simulink model "AccTarSel"  (R2018b)
settings: Solver=FixedStepDiscrete  StartTime=0.0  StopTime=inf  FixedStep=0.01  RelTol=1e-3
PostLoadFcn:
  | if any(exist('dsrtsu_mdlpostloadfcn', 'file') ~= 0), dsrtsu_mdlpostloadfcn('Execute', bdroot); end
values from neighbouring files (symbols this model uses):
  P_adtMaxBDC = 1.0    [AccTarSel.sldd]
  P_aFOCApproachIntpAcitve = -0.6    [AccTarSel.sldd]
  P_aFOCApproachIntpEnsure = -1.8    [AccTarSel.sldd]
  P_CutInEnable = 1.0    [AccTarSel.sldd]
  P_dAimMin = 4.5    [AccTarSel.sldd]
  P_dAimMinAVP = 1.5    [AccTarSel.sldd]
  P_dObjDrvOffMax = 5.0    [AccTarSel.sldd]
  P_dObjDrvOffMin = 3.0    [AccTarSel.sldd]
  P_dObjLowHystDecToStop = 4.5    [AccTarSel.sldd]
  P_dObjLowHystDecToStopAVP = 1.5    [AccTarSel.sldd]
  P_dObjUpperHystDecToStop = 5.0    [AccTarSel.sldd]
  P_dResMax = 5.0    [AccTarSel.sldd]
  P_dStandStill = 3.0    [AccTarSel.sldd]
  P_dStandStillMin = 2.0    [AccTarSel.sldd]
  P_dvarYMax4PO = 1.0    [AccTarSel.sldd]
  P_dyCutInThres = 3.6    [AccTarSel.sldd]
  P_facBDCInit = 0.7    [AccTarSel.sldd]
  P_facBDCIterCalc = 0.8    [AccTarSel.sldd]
  P_facFOCNegDiff = 0.3    [AccTarSel.sldd]
  P_facFOCPosDiff = 0.2    [AccTarSel.sldd]
  P_kapHystThres = 0.0005    [AccTarSel.sldd]
  P_PlausIntegDisable = 0.0    [AccTarSel.sldd]
  P_plausMin4PO = 0.5    [AccTarSel.sldd]
  P_probExistMin4PO = 0.8    [AccTarSel.sldd]
  P_StandObjEnable = 0.0    [AccTarSel.sldd]
  P_tAxTrackNegLower = 0.3    [AccTarSel.sldd]
  P_tAxTrackNegUpper = 0.6    [AccTarSel.sldd]
  P_tAxTrackPosLower = 1.0    [AccTarSel.sldd]
  P_tAxTrackPosUpper = 2.0    [AccTarSel.sldd]
  P_tBDCStartFilt = 0.2    [AccTarSel.sldd]
  P_tCSC = 3.5    [AccTarSel.sldd]
  P_tCurvFilt = 0.2    [AccTarSel.sldd]
  P_tCutInFilt = 0.5    [AccTarSel.sldd]
  P_tFiltAxAbsPONegFast = 0.1    [AccTarSel.sldd]
  P_tFiltAxAbsPONegSlow = 0.4    [AccTarSel.sldd]
  P_tFiltAxAbsPOPosFast = 1.2    [AccTarSel.sldd]
  P_tFiltAxAbsPOPosSlow = 2.0    [AccTarSel.sldd]
  P_tFiltAxAbsPOStand = 2.0    [AccTarSel.sldd]
  P_tFiltDAim = 0.1    [AccTarSel.sldd]
  P_tFiltDsd = 0.1    [AccTarSel.sldd]
  P_tFiltSpdLim = 3.0    [AccTarSel.sldd]
  P_tFiltVxAxPOFast = 0.15    [AccTarSel.sldd]
  P_tFiltVxAxPOSlow = 0.25    [AccTarSel.sldd]
  P_tFOCStatAccelFast = 4.0    [AccTarSel.sldd]
  P_tFOCStatAccelSlow = 3.5    [AccTarSel.sldd]
  P_tFOCStatDecelFast = 4.0    [AccTarSel.sldd]
  P_tFOCStatDecelSlow = 3.2    [AccTarSel.sldd]
  P_tMinDrvPhase = 2.0    [AccTarSel.sldd]
  P_tPredObjLeav = 1.2    [AccTarSel.sldd]
  P_tRollingFilt = 0.5    [AccTarSel.sldd]
  P_tRollingFinFilt = 1.0    [AccTarSel.sldd]
  P_tSSCNeg = 4.5    [AccTarSel.sldd]
  P_tSSCPos = 5.5    [AccTarSel.sldd]
  P_tToStop = 5.0    [AccTarSel.sldd]
  P_tToStopInBDC = 6.0    [AccTarSel.sldd]
  P_tToStopTrig = 4.0    [AccTarSel.sldd]
  P_vEgoDecToStop = 3.0    [AccTarSel.sldd]
  P_vEgoLowBDC = 4.0    [AccTarSel.sldd]
  P_vFOCNegDiff = 4.0    [AccTarSel.sldd]
  P_vFOCPosDiff = 5.0    [AccTarSel.sldd]
  P_vFOCStationaryFast = 15.0    [AccTarSel.sldd]
  P_vFOCStationarySlow = 5.0    [AccTarSel.sldd]
  P_vObjDrvOff = 0.5    [AccTarSel.sldd]
  P_vObjLowHystDecToStop = 0.5    [AccTarSel.sldd]
  P_vObjNoStop = 1.0    [AccTarSel.sldd]
  P_vObjReCalc = 1.0    [AccTarSel.sldd]
  P_vObjStop = 0.3    [AccTarSel.sldd]
  P_vObjUpperHystDecToStop = 0.8    [AccTarSel.sldd]
  P_vStandStill = 0.3    [AccTarSel.sldd]
  P_vStandStillHyst = 0.3    [AccTarSel.sldd]
  P_vyCutInThres = 0.5    [AccTarSel.sldd]
libraries: simulink x21, LPFilter x12
(part 8 of 11)

== system AccTarSel/ACC_Target_Selection/Subsystem/ValidObjCalc/TargetPlausCheck ==
  In1 : Inport
  In2 : Inport  Port=2
  In3 : Inport  Port=3
  Bus Selector : BusSelector  OutputSignals=Valid
  Constant : Constant  Value=0  OutDataTypeStr=boolean
  If : If  IfExpression=u1 == 1
  If Action Subsystem : Subsystem  TreatAsAtomicUnit=on
  Merge : Merge
  Subsystem : Subsystem
  Out1 : Outport
  wires:
  Bus Selector/1 -> If/1  "<Valid>"
  In1/1 -> Subsystem/1(fus_objdata_st), Bus Selector/1  "fus_objdata_st"
  In3/1 -> Subsystem/2(VSI_VehState_st)  "VSI_VehState_st"
  In2/1 -> Subsystem/3(plausibility)  "plausibility"
  If/1 -> Subsystem/Action
  If/2 -> If Action Subsystem/Action
  Constant/1 -> If Action Subsystem/1(In1)
  Subsystem/1(Out1) -> Merge/1
  If Action Subsystem/1(Out1) -> Merge/2
  Merge/1 -> Out1/1

== system AccTarSel/RTI Data/RTI Data Store/RTI Data Store/RTI Data Store ==
  RTI Data Store : Subsystem  mask(RTI_DATA_STORE){}
      mask help:
      | RTI Data Store Block. This block is used by RTI to store internal model dependent data. Deleting this block will result in data loss.
      |
      | NEVER DELETE, COPY, OR MODIFY THIS BLOCK!
      mask Help:
      | RTI Data Store Block. This block is used by RTI to store internal model dependent data. Deleting this block will result in data loss.
      | 
      | NEVER DELETE, COPY, OR MODIFY THIS BLOCK!
      mask Display: text(0.5, 0.5, ' ', 'HorizontalAlignment', 'center');

== system AccTarSel/ACC_Control/FollowObjCtrl/FollowObjValid/ApproachingCtrl/If Action Subsystem ==
  In1 : Inport
  Action Port : ActionPort  ActionType=elseif
  Constant2 : Constant  OutDataTypeStr=single
  Out1 : Outport
  Out2 : Outport  Port=2
  wires:
  In1/1 -> Out1/1
  Constant2/1 -> Out2/1

== system AccTarSel/ACC_Control/FollowObjCtrl/FollowObjValid/ApproachingCtrl/If Action Subsystem2 ==
  Action Port : ActionPort  ActionType=then
  Constant1 : Constant  Value=0  OutDataTypeStr=single
  Constant2 : Constant  Value=0  OutDataTypeStr=single
  Out1 : Outport
  Out2 : Outport  Port=2
  wires:
  Constant1/1 -> Out1/1
  Constant2/1 -> Out2/1

== system AccTarSel/ACC_Control/FollowObjCtrl/FollowObjValid/ApproachingCtrl/If Action Subsystem3 ==
  In1 : Inport
  Action Port : ActionPort  ActionType=else
  Constant2 : Constant  Value=2  OutDataTypeStr=single
  Out1 : Outport
  Out2 : Outport  Port=2
  wires:
  In1/1 -> Out1/1
  Constant2/1 -> Out2/1

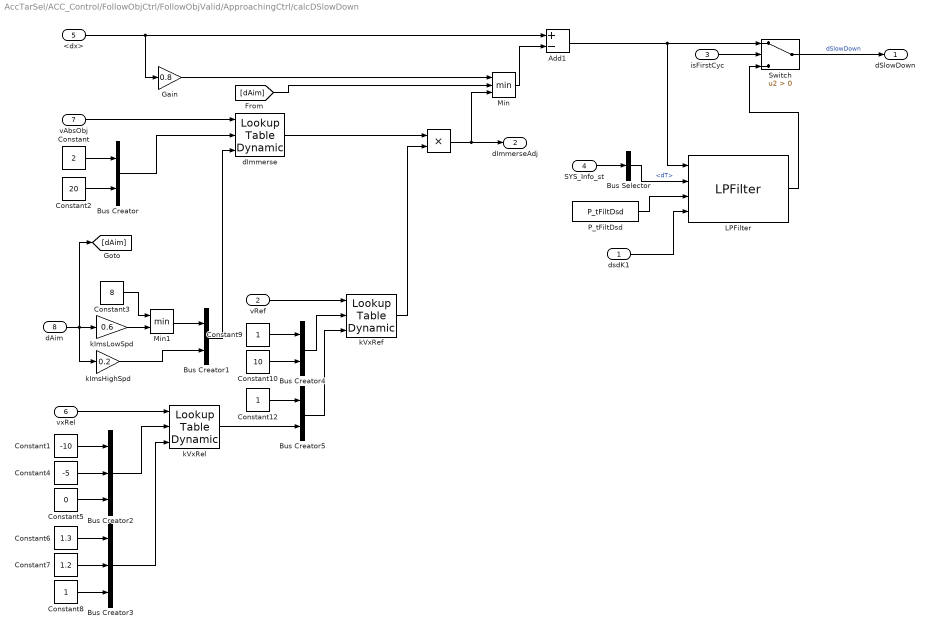
== system AccTarSel/ACC_Control/FollowObjCtrl/FollowObjValid/ApproachingCtrl/calcDSlowDown ==
  dsdK1 : Inport
  vRef : Inport  Port=2
  isFirstCyc : Inport  Port=3
  SYS_Info_st : Inport  Port=4
  <dx> : Inport  Port=5
  vxRel : Inport  Port=6
  vAbsObj : Inport  Port=7
  dAim : Inport  Port=8
  " " : Product
  Add1 : Sum  Inputs=+-
  Bus Creator{,1,4..5} (4 alike) : BusCreator  Inputs=2
  Bus Creator2 : BusCreator  Inputs=3
  Bus Creator3 : BusCreator  Inputs=3
  Bus Selector : BusSelector  OutputSignals=dT
  Constant : Constant  Value=2  OutDataTypeStr=single
  Constant1 : Constant  Value=-10  OutDataTypeStr=single
  Constant10 : Constant  Value=10  OutDataTypeStr=single
  Constant12 : Constant  OutDataTypeStr=single
  Constant2 : Constant  Value=20  OutDataTypeStr=single
  Constant3 : Constant  Value=8  OutDataTypeStr=single
  Constant4 : Constant  Value=-5  OutDataTypeStr=single
  Constant5 : Constant  Value=0  OutDataTypeStr=single
  Constant6 : Constant  Value=1.3  OutDataTypeStr=single
  Constant7 : Constant  Value=1.2  OutDataTypeStr=single
  Constant8 : Constant  OutDataTypeStr=single
  Constant9 : Constant  OutDataTypeStr=single
  Gain : Gain  Gain=0.8
  LPFilter : LPFilter/LPFilter  SystemSampleTime=-1
      settings: SourceProductName=CustomLib
  Min : MinMax  Inputs=3
  Min1 : MinMax  Inputs=2
  P_tFiltDsd : Constant  Value=P_tFiltDsd  OutDataTypeStr=single
  Switch : Switch  Criteria=u2 > Threshold
  dImmerse : simulink/Lookup Tables/Lookup Table Dynamic  LookUpMeth=Interpolation-Use End Values  OutDataType=fixdt('single')  OutScaling=[]  OutputDataTypeScalingMode=Specify via dialog  OutDataTypeStr=single  DoSatur=off
      settings: SourceProductName=Simulink
  kImsHighSpd : Gain  Gain=0.2
  kImsLowSpd : Gain  Gain=0.6
  kVxRef : simulink/Lookup Tables/Lookup Table Dynamic  LookUpMeth=Interpolation-Use End Values  OutDataType=fixdt('single')  OutScaling=[]  OutputDataTypeScalingMode=Specify via dialog  OutDataTypeStr=single  DoSatur=off
      settings: SourceProductName=Simulink
  kVxRel : simulink/Lookup Tables/Lookup Table Dynamic  LookUpMeth=Interpolation-Use End Values  OutDataType=fixdt('single')  OutScaling=[]  OutputDataTypeScalingMode=Specify via dialog  OutDataTypeStr=single  DoSatur=off
      settings: SourceProductName=Simulink
  dSlowDown : Outport
  dImmerseAdj : Outport  Port=2
  wires:
  Min/1 -> Add1/2
  <dx>/1 -> Gain/1, Add1/1
  Gain/1 -> Min/1
  isFirstCyc/1 -> Switch/2
  Add1/1 -> Switch/1, LPFilter/1
  dsdK1/1 -> LPFilter/4
  SYS_Info_st/1 -> Bus Selector/1
  Bus Selector/1 -> LPFilter/2  "<dT>"
  P_tFiltDsd/1 -> LPFilter/3
  LPFilter/1 -> Switch/3
  Switch/1 -> dSlowDown/1  "dSlowDown"
  vAbsObj/1 -> dImmerse/1
  Constant/1 -> Bus Creator/1
  Bus Creator/1 -> dImmerse/2
  dAim/1 -> kImsHighSpd/1, [dAim], kImsLowSpd/1
  [dAim] -> Min/2
  Bus Creator1/1 -> dImmerse/3
  Constant2/1 -> Bus Creator/2
  kImsHighSpd/1 -> Bus Creator1/2
  kImsLowSpd/1 -> Min1/2
  Constant3/1 -> Min1/1
  Min1/1 -> Bus Creator1/1
  vxRel/1 -> kVxRel/1
  Constant4/1 -> Bus Creator2/2
  Constant1/1 -> Bus Creator2/1
  Constant5/1 -> Bus Creator2/3
  Constant8/1 -> Bus Creator3/3
  Constant6/1 -> Bus Creator3/1
  Constant7/1 -> Bus Creator3/2
  Bus Creator2/1 -> kVxRel/2
  Bus Creator3/1 -> kVxRel/3
  Bus Creator5/1 -> kVxRef/3
  Bus Creator4/1 -> kVxRef/2
  kVxRel/1 -> Bus Creator5/2
  Constant12/1 -> Bus Creator5/1
  Constant9/1 -> Bus Creator4/1
  Constant10/1 -> Bus Creator4/2
  vRef/1 -> kVxRef/1
  dImmerse/1 -> " "/1
  kVxRef/1 -> " "/2
  " "/1 -> dImmerseAdj/1, Min/3

== system AccTarSel/ACC_Control/FollowObjCtrl/FollowObjValid/ApproachingCtrl/case1 ==
  vObjRel : Inport
  dSlowDown : Inport  Port=2
  aAbsObj : Inport  Port=3
  Constant2 : Constant  Value=-0.1  OutDataTypeStr=single
  If : If  IfExpression=u1 == 1
  Merge : Merge
  Merge1 : Merge
  Relational Operator : RelationalOperator  Operator=>  OutDataTypeStr=boolean  RndMeth=Simplest
  Subsystem : Subsystem
  Subsystem1 : Subsystem
  tSameSpd : Outport
  aRel : Outport  Port=2
  wires:
  Relational Operator/1 -> If/1
  Constant2/1 -> Relational Operator/2
  dSlowDown/1 -> Subsystem/2(dSlowDown)
  aAbsObj/1 -> Subsystem1/1(aAbsObj), Subsystem/3(aAbsObj)
  Subsystem1/1(tSameSpd) -> Merge/1
  Subsystem/1(tSameSpd) -> Merge/2
  Subsystem/2(aRel) -> Merge1/2
  Subsystem1/2(aRel) -> Merge1/1
  Merge/1 -> tSameSpd/1
  Merge1/1 -> aRel/1
  If/1 -> Subsystem1/Action
  If/2 -> Subsystem/Action
  vObjRel/1 -> Relational Operator/1, Subsystem/1(vObjRel)

== system AccTarSel/ACC_Control/FollowObjCtrl/FollowObjValid/ApproachingCtrl/case2 ==
  vAbsObj : Inport
  vRef : Inport  Port=2
  dSlowDown : Inport  Port=3
  aAbsObj : Inport  Port=4
  Abs : Abs
  Add : Sum
  Constant : Constant  Value=2  OutDataTypeStr=single
  Constant1 : Constant  Value=2  OutDataTypeStr=single
  Constant2 : Constant  Value=-0.1  OutDataTypeStr=single
  Divide : Product  Inputs=*/
  Divide1 : Product  Inputs=*/
  Gain : Gain  Gain=-1
  Min : MinMax  Inputs=2
  Multiply : Product
  Multiply1 : Product
  Square : Math  Operator=square  SaturateOnIntegerOverflow=on
  Square1 : Math  Operator=square  SaturateOnIntegerOverflow=on
  aRelCase2 : Outport
  wires:
  vAbsObj/1 -> Square/1
  Constant/1 -> Multiply/2
  Square/1 -> Divide/1
  Multiply/1 -> Divide/2
  dSlowDown/1 -> Add/1
  vRef/1 -> Square1/1
  Square1/1 -> Divide1/1
  Multiply1/1 -> Divide1/2
  Add/1 -> Multiply1/1
  Constant1/1 -> Multiply1/2
  Divide1/1 -> Gain/1
  Abs/1 -> Multiply/1
  Divide/1 -> Add/2
  Gain/1 -> aRelCase2/1
  aAbsObj/1 -> Min/1
  Min/1 -> Abs/1
  Constant2/1 -> Min/2

== system AccTarSel/ACC_Control/FollowObjCtrl/FollowObjValid/ApproachingCtrl/isObjLeaving ==
  vx : Inport
  isFirstCyc : Inport  Port=2
  ax : Inport  Port=3
  K1 : Inport  Port=4
  AND : Logic  AllPortsSameDT=off  OutDataTypeStr=boolean
  Add : Sum
  Approaching : Subsystem  TreatAsAtomicUnit=on
  Constant : Constant  Value=P_tPredObjLeav
  Constant1 : Constant  Value=-0.2
  Constant2 : Constant  Value=0.2
  Hold : Subsystem  TreatAsAtomicUnit=on
  If : If  NumInputs=2  IfExpression=u1 ==1  ElseIfExpressions=u2 ==1
  Leaving : Subsystem  TreatAsAtomicUnit=on
  Merge : Merge  Inputs=3
  Multiply : Product
  Relational Operator : RelationalOperator  Operator=<=  OutDataTypeStr=boolean  RndMeth=Simplest
  Relational Operator1 : RelationalOperator  OutDataTypeStr=boolean  RndMeth=Simplest
  Relational Operator2 : RelationalOperator  OutDataTypeStr=boolean  RndMeth=Simplest
  Switch : Switch  Criteria=u2 > Threshold
  ObjLeaving : Outport
  wires:
  isFirstCyc/1 -> Switch/2
  vx/1 -> [vx], Add/1
  ax/1 -> [ax], Multiply/1
  Constant/1 -> Multiply/2
  Multiply/1 -> Add/2
  Add/1 -> Relational Operator/1
  Constant1/1 -> Relational Operator/2
  Relational Operator/1 -> If/1, Switch/1
  Constant2/1 -> Relational Operator2/2, Relational Operator1/2
  If/1 -> Approaching/Action
  If/2 -> Leaving/Action
  If/3 -> Hold/Action
  K1/1 -> Hold/1(In1)
  Approaching/1(Out1) -> Merge/1
  Leaving/1(Out1) -> Merge/2
  Hold/1(Out1) -> Merge/3
  Merge/1 -> Switch/3
  Switch/1 -> ObjLeaving/1
  [vx] -> Relational Operator2/1
  [ax] -> Relational Operator1/1
  Relational Operator2/1 -> AND/1
  Relational Operator1/1 -> AND/2
  AND/1 -> If/2

== system AccTarSel/ACC_Control/FollowObjCtrl/FollowObjValid/ApproachingCtrl/tStopObj ==
  note: MotionSts:
      | 0	Unknown
      | 1	Standstill
      | 2	Driving
      | 3	InvDriving
      | 4	Stopped
      | 5	InvStopped
  vAbsObj : Inport
  MotionSts : Inport  Port=2
  aAbsObj : Inport  Port=3
  Abs : Abs
  Constant : Constant  Value=255  OutDataTypeStr=single
  Constant1 : Constant  Value=-0.1  OutDataTypeStr=single
  Constant2 : Constant  OutDataTypeStr=single
  Constant3 : Constant  Value=4  OutDataTypeStr=single
  Constant4 : Constant  Value=0  OutDataTypeStr=single
  Divide : Product  Inputs=*/
  Min : MinMax  Inputs=2
  Min1 : MinMax  Inputs=2
  OR : Logic  Operator=OR  AllPortsSameDT=off  OutDataTypeStr=boolean
  Relational Operator : RelationalOperator  Operator===  OutDataTypeStr=boolean  RndMeth=Simplest
  Relational Operator1 : RelationalOperator  Operator===  OutDataTypeStr=boolean  RndMeth=Simplest
  Switch : Switch  Threshold=0.1
  Switch1 : Switch
  tStopObj : Outport
  wires:
  aAbsObj/1 -> Min1/1, Switch/2
  Constant/1 -> Switch/1, Min/1
  vAbsObj/1 -> Divide/1
  Divide/1 -> Abs/1
  Abs/1 -> Min/2
  Min/1 -> Switch/3
  Constant1/1 -> Min1/2
  Min1/1 -> Divide/2
  MotionSts/1 -> Relational Operator1/1, Relational Operator/1
  Constant2/1 -> Relational Operator/2
  Constant3/1 -> Relational Operator1/2
  Relational Operator/1 -> OR/1
  Relational Operator1/1 -> OR/2
  OR/1 -> Switch1/2
  Constant4/1 -> Switch1/1
  Switch1/1 -> tStopObj/1
  Switch/1 -> Switch1/3

== system AccTarSel/ACC_Control/FollowObjCtrl/FollowObjValid/BrakeDistCtrl/calcA ==
  State : Inport
  Profile : Inport  Port=2
  tElapse : Inport  Port=3
  dRes : Inport  Port=4
  SYS_Info_st : Inport  Port=5
  Constant1 : Constant  Value=3  OutDataTypeStr=single
  Constant3 : Constant  Value=2  OutDataTypeStr=single
  If : If  IfExpression=u1 == 1
  If Action Subsystem : Subsystem  TreatAsAtomicUnit=on
  If Action Subsystem1 : Subsystem  TreatAsAtomicUnit=on
  Merge : Merge
  OR : Logic  Operator=OR  AllPortsSameDT=off  OutDataTypeStr=boolean
  Relational Operator : RelationalOperator  Operator===  OutDataTypeStr=boolean  RndMeth=Simplest
  Relational Operator1 : RelationalOperator  Operator===  OutDataTypeStr=boolean  RndMeth=Simplest
  BDC_Acitve : Outport
  a_BDC : Outport  Port=2
  wires:
  State/1 -> Relational Operator1/1, Relational Operator/1
  Constant3/1 -> Relational Operator/2
  Constant1/1 -> Relational Operator1/2
  Relational Operator/1 -> OR/1
  Relational Operator1/1 -> OR/2
  OR/1 -> BDC_Acitve/1, If/1
  Profile/1 -> If Action Subsystem/1(Profile)
  tElapse/1 -> If Action Subsystem/2(tElapse)
  If/1 -> If Action Subsystem/Action
  If/2 -> If Action Subsystem1/Action
  If Action Subsystem/1(Out1) -> Merge/1
  If Action Subsystem1/1(Out1) -> Merge/2
  Merge/1 -> a_BDC/1
  dRes/1 -> If Action Subsystem/3(dRes)
  SYS_Info_st/1 -> If Action Subsystem/4(SYS_Info_st)

== system AccTarSel/ACC_Control/FollowObjCtrl/FollowObjValid/BrakeDistCtrl/calcCriteria ==
  tElaps : Inport
  BDC_StateK1 : Inport  Port=2
  ProfileK1 : Inport  Port=3
  egoInfo : Inport  Port=4
  objInfo : Inport  Port=5
  Add : Sum
  Bus Selector : BusSelector  OutputSignals=vRef,aRef
  Bus Selector1 : BusSelector  OutputSignals=vx,axAbs,dx
  P_vEgoLowBDC : Constant  Value=P_vEgoLowBDC  OutDataTypeStr=single
  Relational Operator2 : RelationalOperator  Operator=<  OutDataTypeStr=boolean  RndMeth=Simplest
  calcObjStop : Subsystem
  calcProfileReCalc : Subsystem
  ObjToStop : Outport
  ObjToStopTrig : Outport  Port=2
  egoLowSpd : Outport  Port=3
  PreStop : Outport  Port=4
  ProfileReCalc : Outport  Port=5
  dObjToStop : Outport  Port=6
  dRes : Outport  Port=7
  wires:
  objInfo/1 -> Bus Selector1/1
  Bus Selector1/1 -> Add/2  "<vx>"
  Bus Selector1/2 -> calcObjStop/2(aAbsObj)  "<axAbs>"
  Bus Selector/1 -> calcProfileReCalc/2(<vRef>), Add/1, Relational Operator2/1  "<vRef>"
  Bus Selector/2 -> calcProfileReCalc/3(<aRef>)  "<aRef>"
  egoInfo/1 -> Bus Selector/1
  P_vEgoLowBDC/1 -> Relational Operator2/2
  Relational Operator2/1 -> egoLowSpd/1
  Add/1 -> calcProfileReCalc/5(vAbsObj), calcObjStop/1(vAbsObj)  "vAbsObj"
  calcObjStop/1(ObjToStop) -> ObjToStop/1  "ObjToStop"
  calcObjStop/2(ObjToStopTrig) -> ObjToStopTrig/1  "ObjToStopTrig"
  Bus Selector1/3 -> calcProfileReCalc/4(<dx>)  "<dx>"
  calcProfileReCalc/1(ProfileReCalc) -> ProfileReCalc/1
  calcObjStop/3(dObjToStop) -> dObjToStop/1, calcProfileReCalc/1(dObjToStop)
  BDC_StateK1/1 -> calcObjStop/3(BDC_StateK1), calcProfileReCalc/7(BDC_StateK1)
  ProfileK1/1 -> calcProfileReCalc/8(ProfileK1)
  tElaps/1 -> calcProfileReCalc/6(tElaps)
  calcProfileReCalc/2(dRes) -> dRes/1

== system AccTarSel/ACC_Control/FollowObjCtrl/FollowObjValid/BrakeDistCtrl/calcProfile ==
  egoInfo : Inport
  BDC_State : Inport  Port=2
  dObjToStop : Inport  Port=3
  objInfo : Inport  Port=4
  aCvK1 : Inport  Port=5
  Constant1 : Constant  Value=3  OutDataTypeStr=single
  Constant2 : Constant  OutDataTypeStr=single
  Constant3 : Constant  Value=2  OutDataTypeStr=single
  Constant4 : Constant  OutDataTypeStr=single
  If : If  NumInputs=2  IfExpression=u1 == 1  ElseIfExpressions=u2 == 1
  If Action Subsystem : Subsystem  TreatAsAtomicUnit=on
  Memory : Memory
  Memory1 : Memory
  Merge : Merge  Inputs=3
  OR : Logic  Operator=OR  Inputs=3  AllPortsSameDT=off  OutDataTypeStr=boolean
  OR1 : Logic  AllPortsSameDT=off  OutDataTypeStr=boolean
  Relational Operator{,1..3} (4 alike) : RelationalOperator  Operator===  OutDataTypeStr=boolean  RndMeth=Simplest
  calc : Subsystem
  default : Subsystem  TreatAsAtomicUnit=on
  Profile : Outport
  wires:
  dObjToStop/1 -> calc/3(dObjToStop)
  Constant2/1 -> Relational Operator/2
  default/1(default) -> Merge/3
  OR/1 -> If/1
  Memory/1 -> Relational Operator2/1
  calc/1(Profile) -> Merge/1
  If/3 -> default/Action
  egoInfo/1 -> calc/1(egoInfo)
  Relational Operator1/1 -> If/2, OR1/1
  OR1/1 -> OR/2
  Constant4/1 -> Relational Operator2/2
  If/1 -> calc/Action
  objInfo/1 -> calc/2(objInfo)
  Relational Operator2/1 -> OR1/2
  Relational Operator/1 -> OR/1
  Constant3/1 -> Relational Operator1/2
  Merge/1 -> Profile/1, Memory1/1  "Profile"
  Relational Operator3/1 -> OR/3
  BDC_State/1 -> Relational Operator1/1, Relational Operator/1, Relational Operator3/1, Memory/1
  Constant1/1 -> Relational Operator3/2
  If/2 -> If Action Subsystem/Action
  Memory1/1 -> If Action Subsystem/1(In1)
  If Action Subsystem/1(Out1) -> Merge/2
  aCvK1/1 -> calc/4(aCvK1)

== system AccTarSel/ACC_Control/FollowObjCtrl/FollowObjValid/CalcDAim/calcTimeGapToDAim ==
  vRef : Inport
  tTimeGapSet : Inport  Port=2
  1-D Lookup Table : Lookup_n-D  NumberOfTableDimensions=1  BreakpointsForDimension1=[1.4,1.8,2.1]  Table=[1.5,1.4,1.3]  InterpMethod=Flat  InternalRulePriority=Speed  RndMeth=Simplest  InputSameDT=on
  Bus Creator1 : BusCreator  Inputs=2
  Bus Creator2 : BusCreator  Inputs=2
  Constant1 : Constant  OutDataTypeStr=single
  Constant5 : Constant  Value=8.3  OutDataTypeStr=single
  Constant6 : Constant  Value=16.6  OutDataTypeStr=single
  "GainTimeGap " : simulink/Lookup Tables/Lookup Table Dynamic  LookUpMeth=Interpolation-Use End Values  OutDataType=fixdt('single')  OutScaling=[]  OutputDataTypeScalingMode=Specify via dialog  OutDataTypeStr=single  DoSatur=off
      settings: SourceProductName=Simulink
  Multiply : Product
  tTimeGapAct : Product
  dAimTimeGap : Outport
  wires:
  vRef/1 -> Multiply/1, "GainTimeGap "/1
  Bus Creator2/1 -> "GainTimeGap "/2
  Constant6/1 -> Bus Creator2/2
  Constant5/1 -> Bus Creator2/1
  Constant1/1 -> Bus Creator1/1
  1-D Lookup Table/1 -> Bus Creator1/2
  Bus Creator1/1 -> "GainTimeGap "/3
  tTimeGapSet/1 -> tTimeGapAct/2, 1-D Lookup Table/1
  "GainTimeGap "/1 -> tTimeGapAct/1
  tTimeGapAct/1 -> Multiply/2
  Multiply/1 -> dAimTimeGap/1

== system AccTarSel/ACC_Control/FollowObjCtrl/FollowObjValid/FOC_MIX/Subsystem ==
  In1 : Inport
  In2 : Inport  Port=2
  If : If  NumInputs=2  IfExpression=u1 == 1  ElseIfExpressions=u2 == 1
  If Action Subsystem : Subsystem  TreatAsAtomicUnit=on
  If Action Subsystem1 : Subsystem  TreatAsAtomicUnit=on
  If Action Subsystem2 : Subsystem  TreatAsAtomicUnit=on
  Logical Operator : Logic  Operator=OR  AllPortsSameDT=off  OutDataTypeStr=boolean
  Merge : Merge  Inputs=3
  P_aFOCApproachIntpAcitve : Constant  Value=P_aFOCApproachIntpAcitve
  P_aFOCApproachIntpEnsure : Constant  Value=P_aFOCApproachIntpEnsure
  Relational Operator : RelationalOperator  Operator=<=  OutDataTypeStr=boolean  RndMeth=Simplest
  Relational Operator1 : RelationalOperator  Operator=<=  OutDataTypeStr=boolean  RndMeth=Simplest
  Relational Operator2 : RelationalOperator  Operator=>  OutDataTypeStr=boolean  RndMeth=Simplest
  aFocMix : Outport
  wires:
  If/3 -> If Action Subsystem2/Action
  If/1 -> If Action Subsystem/Action
  Relational Operator2/1 -> If/2
  If Action Subsystem/1(Out1) -> Merge/1
  In1/1 -> If Action Subsystem1/1(aStat), If Action Subsystem/1(aStat), If Action Subsystem2/1(aStat), Relational Operator/1
  Relational Operator/1 -> Logical Operator/1
  If Action Subsystem1/1(Out1) -> Merge/2
  In2/1 -> If Action Subsystem/2(aApprh), If Action Subsystem2/2(aApprh), Relational Operator2/1, Relational Operator1/1
  P_aFOCApproachIntpAcitve/1 -> If Action Subsystem2/3(aActive), Relational Operator2/2, Relational Operator/2
  P_aFOCApproachIntpEnsure/1 -> If Action Subsystem2/4(aEnsure), Relational Operator1/2
  Logical Operator/1 -> If/1
  If/2 -> If Action Subsystem1/Action
  Relational Operator1/1 -> Logical Operator/2
  If Action Subsystem2/1(Out1) -> Merge/3
  Merge/1 -> aFocMix/1  "aFocMix"

== system AccTarSel/ACC_Control/FollowObjCtrl/FollowObjValid/StationaryCtrl/If Action Subsystem1 ==
  vRelAim : Inport
  vRel : Inport  Port=2
  Action Port : ActionPort  ActionType=then
  Add : Sum  Inputs=+-
  Out1 : Outport
  wires:
  vRelAim/1 -> Add/1
  vRel/1 -> Add/2
  Add/1 -> Out1/1
